simulink model "plant_1"  (R2023b)
settings: Solver=VariableStepAuto  StartTime=0.0  StopTime=10  FixedStep=10e-5
settings Model: Creator=Mehmet  LastModifiedBy=misca
settings SolverCC: AlgebraicLoopSolver=TrustRegion
settings DataIOCC: ReturnWorkspaceOutputs=off
settings DebuggingCC: UnconnectedInputMsg=warning  UnconnectedOutputMsg=warning  UnconnectedLineMsg=warning  ArithmeticOperatorsInVariantConditions=warning
settings ModelReferenceCC: EnableRefExpFcnMdlSchedulingChecks=on
settings SFSimCC: SimUseLocalCustomCode=off  CustomCodeUndefinedFunction=UseInterfaceOnly
settings RTWCC: RTWUseLocalCustomCode=off

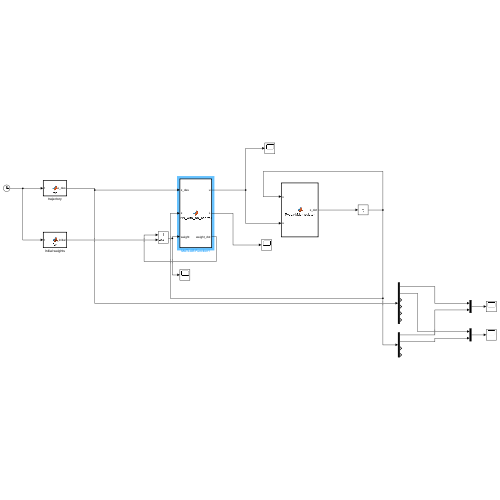
[thumbnail: Simulink's stored preview of the top-level diagram]
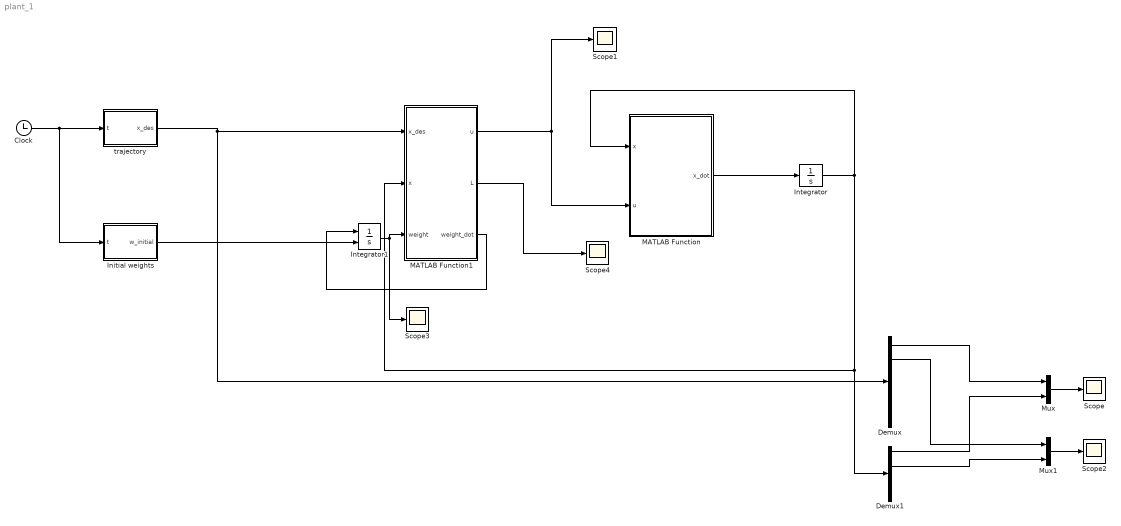
== system plant_1 ==
  Clock : Clock
  Demux : Demux  Outputs=6
  Demux1 : Demux
  Initial weights : MATLAB Function  TreatAsAtomicUnit=on
  Integrator : Integrator  InitialCondition=[0;0;0;0]
  Integrator1 : Integrator  InitialConditionSource=external  InitialCondition=[0;0]
  MATLAB Function : MATLAB Function  TreatAsAtomicUnit=on
  MATLAB Function1 : MATLAB Function  TreatAsAtomicUnit=on
  Mux : Mux  Inputs=2
  Mux1 : Mux  Inputs=2
  Scope{,1..4} (5 alike) : Scope
  trajectory : MATLAB Function  TreatAsAtomicUnit=on
  wires:
  MATLAB Function1/1(u) -> MATLAB Function/2(u), Scope1/1
  Clock/1 -> Initial weights/1(t), trajectory/1(t)
  trajectory/1(x_des) -> MATLAB Function1/1(x_des), Demux/1
  Demux/1 -> Mux/1
  Demux1/1 -> Mux/2
  Mux/1 -> Scope/1
  MATLAB Function/1(x_dot) -> Integrator/1
  Integrator/1 -> MATLAB Function1/2(x), Demux1/1, MATLAB Function/1(x)
  Mux1/1 -> Scope2/1
  Demux/2 -> Mux1/1
  Demux1/2 -> Mux1/2
  MATLAB Function1/3(weight_dot) -> Integrator1/1
  Integrator1/1 -> Scope3/1, MATLAB Function1/3(weight)
  MATLAB Function1/2(L) -> Scope4/1
  Initial weights/1(w_initial) -> Integrator1/2

== matlab function plant_1/MATLAB Function1 ==
  data: x_des input; u output; L output; x input; weight input; weight_dot output
function [u,L,weight_dot]  = FLNN_with_nn_controller(x_des,x,weight)

g= 9.81; % arm parameters
 
Kv = 20*eye(2); % controller parameters
lam = 5*eye(2);

% tracking errors
qd = x_des(1:2,1);
qdp = x_des(3:4,1);
qdpp = x_des(5:6,1);

e = qd - [x(1) x(2)]';
ep = qdp - [x(3) x(4)]';

r = ep + lam*e;

zeta1 = qdpp + lam*ep;
zeta2 = qdp + lam*e;

%%%%%%%%%%%%%%%%%%%%%%%%%%%%%%%%%%%%%%%%%%%%%%%%%%%%%%%%%%
%% FLNN application
H = 4;
K = 2;

w = weight;

x_m_q = [zeta1'.*1,   zeta1'.*sin(x(1:2)'),    zeta1'.*cos(x(1:2)')];
x_v_m = [zeta2'.*sin(x(1:2)').*x(3:4)',  zeta2'.*cos(x(1:2)').*x(3:4)'];
x_g_q = [cos(x(1:2)'),   sin(x(1:2)'),   sin(x(1:2)').*cos(x(1:2)'),   cos(x(1:2)').*cos(x(1:2)')];
x_f_qd = [x(3:4)',   sign(x(3:4)')];

phi_x = zeros(H,1);

phi_x(1,1) = sum(x_m_q);
phi_x(2,1) = sum(x_v_m);
phi_x(3,1) = sum(x_g_q);
phi_x(4,1) = sum(x_f_qd);

tau = zeros(K,1);

for k = 1 : 1 : K
   
    cont_in = 0;
    
    for h = 1 : 1 : H
        
        cont_in = cont_in + w(h,k)*phi_x(h,1);
        
    end
    
    tau(k) = cont_in;
    
end


%% training function

w_dot = zeros(size(w));

% learning rate
F = 50;

for k = 1 : 1 : K
    
    for h = 1 : 1 : H
   
        w_dot(h,k) = F*phi_x(h,1)*r(k);
        
    end
    
end


%% FLNN application
%%%%%%%%%%%%%%%%%%%%%%%%%%%%%%%%%%%%%%%%%%%%%%%%%%%%%%%%%%

weight_dot = w_dot;

u = tau + Kv*r;

L = 1/2*r'*r;


end

== matlab function plant_1/MATLAB Function ==
  data: x input; u input; x_dot output
function x_dot = TwoLinkManipulator(x,u)

% arm parameters
m1 = 0.8; 
m2 = 2.3; 
a1 = 1; 
a2 = 1; 
g = 9.81;   

% inertia M(q) and nonlinear terms N(q,qdot)
M11= (m1 + m2)*a1^2 + m2*a2^2 + 2*m2*a1*a2*cos(x(2)) ;
M12= m2*a2^2 + m2*a1*a2*cos(x(2)) ;
M22= m2*a2^2 ;
N1= -m2*a1*a2*(2*x(3)*x(4) + x(4)^2)*sin(x(2)) ;
N1= N1 + (m1 + m2)*g*a1*cos(x(1)) + m2*g*a2*cos(x(1) + x(2));
N2= m2*a1*a2*x(3)^2*sin(x(2)) + m2*g*a2*cos(x(1) + x(2)) ;

% Inversion of M(q) (for large values of n, use least-squares)
det= M11*M22 - M12*M12 ;
MI11= M22/det ;
MI12= -M12/det ;
MI22= M11/det ;

tau = zeros(2,1);

tau = u;
%% control input
tau1 = tau(1,1);
tau2 = tau(2,1);

q = zeros(4,1);

q(1) = x(3);
q(2) = x(4);
q(3) = MI11*(-N1 + tau1) + MI12*(-N2 + tau2);
q(4) = MI12*(-N1 + tau1) + MI22*(-N2 + tau2);

x_dot = q;

end

== matlab function plant_1/trajectory ==
  data: t input; x_des output
function x_des = fcn(t)

% compute desired trajectory
period= 1 ; amp1= 1 ; amp2= 1 ;
fact= 2*pi/period;
sinf= sin(fact*t);
cosf= cos(fact*t);
qd= [amp1*sinf amp2*cosf];
qdp= fact*[amp1*cosf -amp2*sinf];
qdpp= -fact^2*qd;

x_des = [qd qdp qdpp]';

end

== matlab function plant_1/Initial weights ==
  data: t input; w_initial output
function w_initial = fcn(t)

H = 4;
K = 2;

w = zeros(H,K);

w_initial = w;


end
